simulink model "gm_ControllerTestbench"  (R2020b)
settings: Solver=VariableStepAuto  StartTime=0.0  StopTime=4  RelTol=1e-3
model workspace (MAT data in the model file):
  randSeedTorque = 0
  randomSeedSpeed = 0
undefined symbols (not defined in the file or in its folder): DiscIntNeverNeededParam, I_max, Position_PI_Limit
libraries: simulink x4, hdlmdlgenlib x1
(part 1 of 2)
settings Model: Creator=ciaran  LastModifiedBy=ciaran
settings OptimizationCC: BlockReduction=off  ConditionallyExecuteInputs=off
settings DebuggingCC: InheritedTsInSrcMsg=none

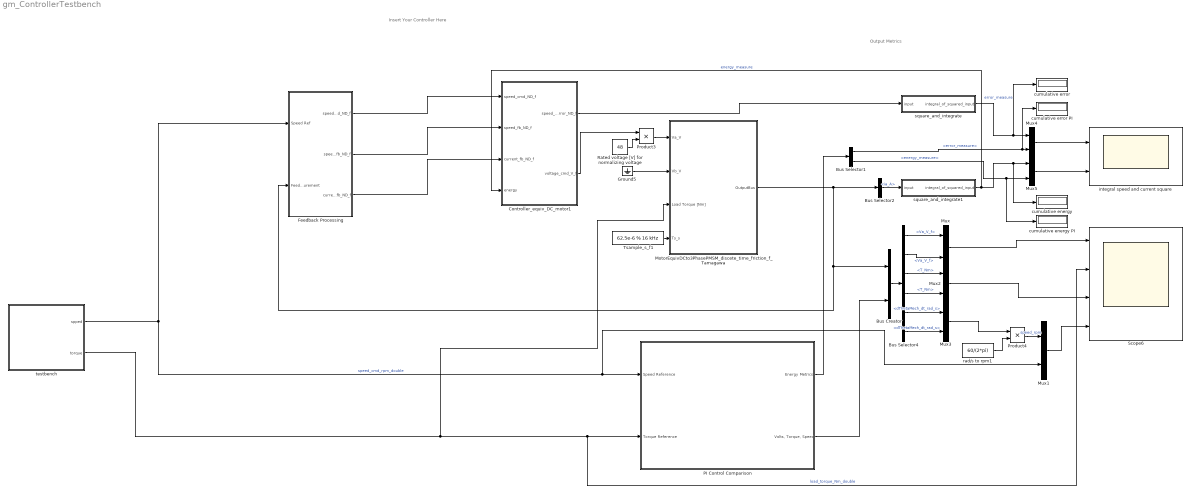
== system gm_ControllerTestbench ==
  note: Insert Your Controller Here
  note: Output Metrics
  Bus Creator : BusCreator  Inputs=2
  Bus Selector1 : BusSelector  OutputSignals=error_measure,energy_measure
  Bus Selector2 : BusSelector  OutputSignals=ia_A
  Bus Selector4 : BusSelector  OutputSignals=signal1.Va_V_f,signal2.Va_V_f,signal1.T_Nm,signal2.T_Nm,signal1.dThetaMech_dt_rad_s,signal2.dThetaMech_dt_rad_s
  Controller_equiv_DC_motor1 : Subsystem
  Feedback Processing : Subsystem
  Ground5 : Ground
  MotorEquivDCto3PhasePMSM_discete_time_friction_f_Tamagawa : Subsystem  mask(Intel PMSM equiv DC){R_ohm=0.68/3, L_H=3e-3/3, Ke_Vs_rad=0.07, Kt_Nm_A=0.07, PolePairs_int=2, J_kgm2=0.165e-4, Tf_Nm=0.02}
      mask prompts: R_ohm "Phase resistance [Ohm]"; L_H "Phase inductance [H]"; Ke_Vs_rad "Back-emf constant kE, based on peak phase values [Vs/rad]"; Kt_Nm_A "Motor torque constant kT, based on peak phase values [Nm/A]"; PolePairs_int "Number of pole pairs (0.5*n poles)  [integer]"; J_kgm2 "Mechanical inertia [kgm^2]"; Tf_Nm "Static friction Tf [Nm]"
      mask help: Intel motor model, equiv DC to PMSM
  Mux{,1..5} (6 alike) : Mux  Inputs=2
  PI Control Comparison : Subsystem
  Product3 : Product
  Product4 : Product
  Rated voltage [V] for normalizing voltage : Constant  Value=48  OutDataTypeStr=double
  Scope6 : Scope  NumInputPorts=4
  Tsample_s_f1 : Constant  Value=62.5e-6 % 16 kHz  OutDataTypeStr=double
  cumulative energy : Display
  cumulative energy PI : Display
  cumulative error : Display
  cumulative error PI : Display
  integral speed and current square : Scope  NumInputPorts=2
  rad/s to rpm1 : Constant  Value=60/(2*pi)  OutDataTypeStr=double
  square_and_integrate : Subsystem
  square_and_integrate1 : Subsystem
  testbench : Subsystem
  wires:
  Bus Selector2/1 -> square_and_integrate1/1(input)  "<ia_A>"
  Ground5/1 -> MotorEquivDCto3PhasePMSM_discete_time_friction_f_Tamagawa/2(Vb_V)
  Tsample_s_f1/1 -> MotorEquivDCto3PhasePMSM_discete_time_friction_f_Tamagawa/4(Ts_s)
  rad/s to rpm1/1 -> Product4/2
  square_and_integrate1/1(integral_of_squared_input) -> Controller_equiv_DC_motor1/4(energy), cumulative energy/1, Mux5/1  "energy_measure"
  Controller_equiv_DC_motor1/1(speed_error_ND_f) -> square_and_integrate/1(input)
  MotorEquivDCto3PhasePMSM_discete_time_friction_f_Tamagawa/1(OutputBus) -> Feedback Processing/2(Feedback Measurement), Bus Creator/1, Bus Selector2/1
  square_and_integrate/1(integral_of_squared_input) -> Mux4/1, cumulative error/1  "error_measure"
  testbench/1(spped) -> Mux1/2, PI Control Comparison/1(Speed Reference), Feedback Processing/1(Speed Ref)  "speed_cmd_rpm_double"
  testbench/2(torque) -> MotorEquivDCto3PhasePMSM_discete_time_friction_f_Tamagawa/3(Load Torque [Nm]), Scope6/2, PI Control Comparison/2(Torque Reference)  "load_torque_Nm_double"
  Feedback Processing/1(speed_cmd_ND_f) -> Controller_equiv_DC_motor1/1(speed_cmd_ND_f)
  Feedback Processing/2(speed_fb_ND_f) -> Controller_equiv_DC_motor1/2(speed_fb_ND_f)
  Feedback Processing/3(current_fb_ND_f) -> Controller_equiv_DC_motor1/3(current_fb_ND_f)
  PI Control Comparison/2("Volts, Torque, Speed") -> Bus Creator/2
  Bus Creator/1 -> Bus Selector4/1
  Bus Selector4/1 -> Mux/1  "<Va_V_f>"
  Bus Selector4/2 -> Mux/2  "<Va_V_f>"
  Bus Selector4/3 -> Mux2/1  "<T_Nm>"
  Bus Selector4/4 -> Mux2/2  "<T_Nm>"
  Mux2/1 -> Scope6/3
  Mux3/1 -> Product4/1
  PI Control Comparison/1(Energy Metrics) -> Bus Selector1/1
  Mux4/1 -> integral speed and current square/1
  Bus Selector1/1 -> cumulative error PI/1, Mux4/2  "<error_measure>"
  Mux5/1 -> integral speed and current square/2
  Bus Selector1/2 -> cumulative energy PI/1, Mux5/2  "<energy_measure>"
  Rated voltage [V] for normalizing voltage/1 -> Product3/2
  Controller_equiv_DC_motor1/2(voltage_cmd_V_f) -> Product3/1
  Product3/1 -> MotorEquivDCto3PhasePMSM_discete_time_friction_f_Tamagawa/1(Va_V)
  Product4/1 -> Mux1/1  "speed_rpm"
  Mux1/1 -> Scope6/4
  Mux/1 -> Scope6/1
  Bus Selector4/5 -> Mux3/1  "<dThetaMech_dt_rad_s>"
  Bus Selector4/6 -> Mux3/2  "<dThetaMech_dt_rad_s>"

== system gm_ControllerTestbench/Controller_equiv_DC_motor1 ==
  note: RL Controller
  speed_cmd_ND_f : Inport
  speed_fb_ND_f : Inport  Port=2  PortDimensions=1
  current_fb_ND_f : Inport  Port=3  PortDimensions=1
  energy : Inport  Port=4
  1 to reset : ManualSwitch
  FALSE_bool : Constant  Value=0  OutDataTypeStr=boolean
  PI_Ctrl_float_speed : Subsystem
  TRUE_bool : Constant  OutDataTypeStr=boolean
  abs_limit_output_ND_f : Constant  OutDataTypeStr=double
  speed_error_ND_f : Outport
  voltage_cmd_V_f : Outport  Port=2
  wires:
  speed_cmd_ND_f/1 -> PI_Ctrl_float_speed/1(cmd_f)
  speed_fb_ND_f/1 -> PI_Ctrl_float_speed/2(fb_f)
  abs_limit_output_ND_f/1 -> PI_Ctrl_float_speed/3(output_abs_limit_f)
  current_fb_ND_f/1 -> PI_Ctrl_float_speed/6(Icurrent_fb)
  1 to reset/1 -> PI_Ctrl_float_speed/4(Reset_bool)
  FALSE_bool/1 -> 1 to reset/1
  TRUE_bool/1 -> 1 to reset/2
  PI_Ctrl_float_speed/1(error_f) -> speed_error_ND_f/1  "speed_error_ND_f"
  energy/1 -> PI_Ctrl_float_speed/5(energy)
  PI_Ctrl_float_speed/2(output_f) -> voltage_cmd_V_f/1

== system gm_ControllerTestbench/Feedback Processing ==
  note: Constant Parameters
  note: Feedback Variables (Observations)
  Speed Ref : Inport
  Feedback Measurement : Inport  Port=2
  Bus Selector1 : BusSelector  OutputSignals=dThetaMech_dt_rad_s,ia_A
  Delay_current_measure : Delay  DelayLength=1  InitialCondition=0
  Delay_speed_measure : Delay  InitialCondition=0
  Inverse ated current [A] for normalizing current : Constant  Value=1/5.7  OutDataTypeStr=double
  Inverse rated speed [1/rpm] for normalizing speed : Constant  Value=1/5000  OutDataTypeStr=double
  Product : Product
  Product1 : Product  Inputs=***
  Product2 : Product
  rad/s to rpm : Constant  Value=60/(2*pi)  OutDataTypeStr=double
  speed_cmd_ND_f : Outport
  speed_fb_ND_f : Outport  Port=2
  current_fb_ND_f : Outport  Port=3
  wires:
  Speed Ref/1 -> Product/1
  Feedback Measurement/1 -> Bus Selector1/1
  Inverse ated current [A] for normalizing current/1 -> Product2/2  "speed_cmd_rpm_double"
  Delay_current_measure/1 -> current_fb_ND_f/1
  rad/s to rpm/1 -> Product1/2
  Product/1 -> speed_cmd_ND_f/1  "speed_cmd_ND_f"
  Product1/1 -> Delay_speed_measure/1  "speed_fb_ND_f"
  Bus Selector1/2 -> Product2/1  "<ia_A>"
  Bus Selector1/1 -> Product1/3  "<dThetaMech_dt_rad_s>"
  Delay_speed_measure/1 -> speed_fb_ND_f/1
  Product2/1 -> Delay_current_measure/1  "current_fb_ND_f"
  Inverse rated speed [1/rpm] for normalizing speed/1 -> Product1/1, Product/2

== system gm_ControllerTestbench/MotorEquivDCto3PhasePMSM_discete_time_friction_f_Tamagawa ==
  Va_V : Inport
  Vb_V : Inport  Port=2
  Load Torque [Nm] : Inport  Port=3
  Ts_s : Inport  Port=4
  Bus Creator1 : BusCreator  Inputs=7
  Load Torque [Nm]1 : InportShadow  Port=3
  Motor electromagnetic : Subsystem
  Motor mechanical : Subsystem  mask(Inertia){J_kgm2=J_kgm2}
      mask prompts: J_kgm2 "Inertia [kgm^2]"
      mask help:
      | Mechanical inertia with two attachment points A and B.
      | Torque is applied to the inertia from side A and side B.
      | The combined torque acting on the inertia produces acceleration,
      | velocity and displacement. Velocity and displacement are output as these
      | are the states of the system.
  Ts_s1 : InportShadow  Port=4
  Va_V1 : InportShadow
  Vb_V1 : InportShadow  Port=2
  OutputBus : Outport
  wires:
  Ts_s1/1 -> Motor electromagnetic/4(Ts_s)
  Motor mechanical/1(dTheta_dt_rad_s) -> Motor electromagnetic/3(dThetaMech_dt_rad_s), Bus Creator1/6  "dThetaMech_dt_rad_s"
  Ts_s/1 -> Motor mechanical/3(Ts_s)
  Load Torque [Nm]/1 -> Motor mechanical/2(TB_Nm)  "TL_Nm_f"
  Va_V/1 -> Motor electromagnetic/1(Va_V)  "Va_V_f"
  Bus Creator1/1 -> OutputBus/1
  Vb_V/1 -> Motor electromagnetic/2(Vb_V)  "Vb_V_f"
  Va_V1/1 -> Bus Creator1/1  "Va_V_f"
  Vb_V1/1 -> Bus Creator1/2  "Vb_V_f"
  Motor electromagnetic/1(ia_A) -> Bus Creator1/4  "ia_A"
  Motor electromagnetic/2(T_Nm) -> Motor mechanical/1(TA_Nm), Bus Creator1/5  "T_Nm"
  Motor mechanical/2(Theta_rad) -> Bus Creator1/7  "ThetaMech_rad"
  Load Torque [Nm]1/1 -> Bus Creator1/3  "TL_Nm_f"

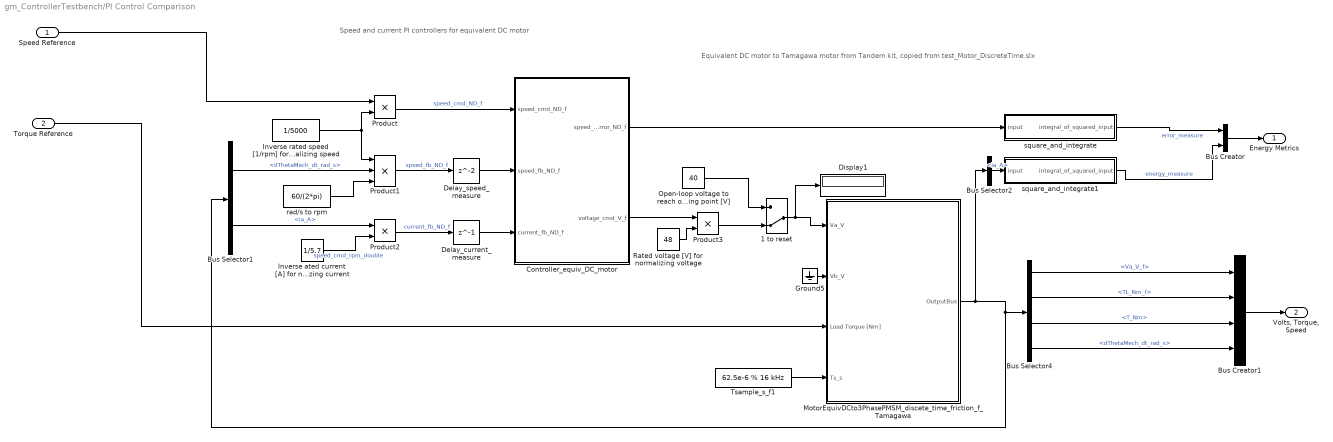
== system gm_ControllerTestbench/PI Control Comparison ==
  note: Speed and current PI controllers
      | for equivalent DC motor
  note: Equivalent DC motor to Tamagawa motor from Tandem kit,
      | copied from test_Motor_DiscreteTime.slx
  Speed Reference : Inport
  Torque Reference : Inport  Port=2
  1 to reset : ManualSwitch  CurrentSetting=0
  Bus Creator : BusCreator  Inputs=2
  Bus Creator1 : BusCreator  Inputs=4
  Bus Selector1 : BusSelector  OutputSignals=dThetaMech_dt_rad_s,ia_A
  Bus Selector2 : BusSelector  OutputSignals=ia_A
  Bus Selector4 : BusSelector  OutputSignals=Va_V_f,TL_Nm_f,T_Nm,dThetaMech_dt_rad_s
  Controller_equiv_DC_motor : Subsystem
  Delay_current_measure : Delay  DelayLength=1  InitialCondition=0
  Delay_speed_measure : Delay  InitialCondition=0
  Display1 : Display
  Ground5 : Ground
  Inverse ated current [A] for normalizing current : Constant  Value=1/5.7  OutDataTypeStr=double
  Inverse rated speed [1/rpm] for normalizing speed : Constant  Value=1/5000  OutDataTypeStr=double
  MotorEquivDCto3PhasePMSM_discete_time_friction_f_Tamagawa : Subsystem  mask(Intel PMSM equiv DC){R_ohm=0.68/3, L_H=3e-3/3, Ke_Vs_rad=0.07, Kt_Nm_A=0.07, PolePairs_int=2, J_kgm2=0.165e-4, Tf_Nm=0.02}
      mask prompts: R_ohm "Phase resistance [Ohm]"; L_H "Phase inductance [H]"; Ke_Vs_rad "Back-emf constant kE, based on peak phase values [Vs/rad]"; Kt_Nm_A "Motor torque constant kT, based on peak phase values [Nm/A]"; PolePairs_int "Number of pole pairs (0.5*n poles)  [integer]"; J_kgm2 "Mechanical inertia [kgm^2]"; Tf_Nm "Static friction Tf [Nm]"
      mask help: Intel motor model, equiv DC to PMSM
  Open-loop voltage to reach operating point [V] : Constant  Value=40  OutDataTypeStr=double
  Product : Product
  Product1 : Product  Inputs=***
  Product2 : Product
  Product3 : Product
  Rated voltage [V] for normalizing voltage : Constant  Value=48  OutDataTypeStr=double
  Tsample_s_f1 : Constant  Value=62.5e-6 % 16 kHz  OutDataTypeStr=double
  rad/s to rpm : Constant  Value=60/(2*pi)  OutDataTypeStr=double
  square_and_integrate : Subsystem
  square_and_integrate1 : Subsystem
  Energy Metrics : Outport
  "Volts, Torque, Speed" : Outport  Port=2
  wires:
  Open-loop voltage to reach operating point [V]/1 -> 1 to reset/1
  Delay_speed_measure/1 -> Controller_equiv_DC_motor/2(speed_fb_ND_f)
  Ground5/1 -> MotorEquivDCto3PhasePMSM_discete_time_friction_f_Tamagawa/2(Vb_V)
  Tsample_s_f1/1 -> MotorEquivDCto3PhasePMSM_discete_time_friction_f_Tamagawa/4(Ts_s)
  Controller_equiv_DC_motor/2(voltage_cmd_V_f) -> Product3/1
  Inverse ated current [A] for normalizing current/1 -> Product2/2  "speed_cmd_rpm_double"
  Controller_equiv_DC_motor/1(speed_error_ND_f) -> square_and_integrate/1(input)
  Rated voltage [V] for normalizing voltage/1 -> Product3/2
  square_and_integrate1/1(integral_of_squared_input) -> Bus Creator/2  "energy_measure"
  Bus Selector1/2 -> Product2/1  "<ia_A>"
  Delay_current_measure/1 -> Controller_equiv_DC_motor/3(current_fb_ND_f)
  Bus Selector1/1 -> Product1/2  "<dThetaMech_dt_rad_s>"
  rad/s to rpm/1 -> Product1/3
  Product2/1 -> Delay_current_measure/1  "current_fb_ND_f"
  Product3/1 -> 1 to reset/2
  Bus Selector2/1 -> square_and_integrate1/1(input)  "<ia_A>"
  Inverse rated speed [1/rpm] for normalizing speed/1 -> Product/2, Product1/1
  MotorEquivDCto3PhasePMSM_discete_time_friction_f_Tamagawa/1(OutputBus) -> Bus Selector2/1, Bus Selector1/1, Bus Selector4/1
  1 to reset/1 -> Display1/1, MotorEquivDCto3PhasePMSM_discete_time_friction_f_Tamagawa/1(Va_V)
  Product1/1 -> Delay_speed_measure/1  "speed_fb_ND_f"
  Product/1 -> Controller_equiv_DC_motor/1(speed_cmd_ND_f)  "speed_cmd_ND_f"
  square_and_integrate/1(integral_of_squared_input) -> Bus Creator/1  "error_measure"
  Torque Reference/1 -> MotorEquivDCto3PhasePMSM_discete_time_friction_f_Tamagawa/3(Load Torque [Nm])
  Speed Reference/1 -> Product/1
  Bus Selector4/1 -> Bus Creator1/1  "<Va_V_f>"
  Bus Selector4/2 -> Bus Creator1/2  "<TL_Nm_f>"
  Bus Selector4/3 -> Bus Creator1/3  "<T_Nm>"
  Bus Selector4/4 -> Bus Creator1/4  "<dThetaMech_dt_rad_s>"
  Bus Creator/1 -> Energy Metrics/1
  Bus Creator1/1 -> "Volts, Torque, Speed"/1

== system gm_ControllerTestbench/square_and_integrate ==
  input : Inport
  Add : Sum
  Product6 : Product  Inputs=***
  Tsample_s_f2 : Constant  Value=62.5e-6 % 16 kHz  OutDataTypeStr=double
  delay_to_integrate : Delay  DelayLength=1  InitialCondition=0
  integral_of_squared_input : Outport
  wires:
  delay_to_integrate/1 -> integral_of_squared_input/1, Add/2
  Product6/1 -> Add/1
  Tsample_s_f2/1 -> Product6/3
  Add/1 -> delay_to_integrate/1
  input/1 -> Product6/1, Product6/2

== system gm_ControllerTestbench/square_and_integrate1 ==
  input : Inport
  Add : Sum
  Product6 : Product  Inputs=***
  Tsample_s_f2 : Constant  Value=62.5e-6 % 16 kHz  OutDataTypeStr=double
  delay_to_integrate : Delay  DelayLength=1  InitialCondition=0
  integral_of_squared_input : Outport
  wires:
  input/1 -> Product6/2, Product6/1
  Add/1 -> delay_to_integrate/1
  Tsample_s_f2/1 -> Product6/3
  Product6/1 -> Add/1
  delay_to_integrate/1 -> Add/2, integral_of_squared_input/1

== system gm_ControllerTestbench/testbench ==
  Constant : Constant  Value=5000
  Gain : Gain  Gain=0.38
  Rate Transition2 : RateTransition  OutPortSampleTime=62.5e-6
  Rate Transition3 : RateTransition  OutPortSampleTime=62.5e-6
  Repeating Sequence Stair : simulink/Sources/Repeating Sequence Stair  OutValues="[5000 -5000 5000 0  0 100 0 -100 -1500 1500 200 -200 3000 -3000 -4000 4000 0 10 20 0 -10 -20].'"  tsamp=3500*62.5e-6  OutMin=[]  OutMax=[]  OutDataTypeStr=double  OutputDataTypeScalingMode=double  OutDataType=fixdt(0,8)  ConRadixGroup=Best Precision: Vector-wise  OutScaling=2^-12
  Repeating Sequence Stair1 : simulink/Sources/Repeating Sequence Stair  OutValues=[1 -1 0 0.5 -0.5].'  tsamp=875*62.5e-6  OutMin=[]  OutMax=[]  OutDataTypeStr=double  OutputDataTypeScalingMode=double  OutDataType=fixdt(0,8)  ConRadixGroup=Best Precision: Vector-wise  OutScaling=2^-12
  spped : Outport
  torque : Outport  Port=2
  wires:
  Rate Transition3/1 -> torque/1  "speed_cmd_rpm_double"
  Repeating Sequence Stair/1 -> Rate Transition2/1
  Repeating Sequence Stair1/1 -> Gain/1
  Gain/1 -> Rate Transition3/1
  Constant/1 -> spped/1

== system gm_ControllerTestbench/Controller_equiv_DC_motor1/PI_Ctrl_float_speed ==
  note: Error Input
  cmd_f : Inport
  fb_f : Inport  Port=2
  output_abs_limit_f : Inport  Port=3
  Reset_bool : Inport  Port=4
  energy : Inport  Port=5
  Icurrent_fb : Inport  Port=6
  Constant1 : Constant  Value=0  OutDataTypeStr=Inherit: Inherit via back propagation
  Reinforcement Learning1 : Subsystem
  Subtract1 : Sum  Inputs=+-
  Unit Delay1 : UnitDelay  SampleTime=-1  HasFrameUpgradeWarning=on
  limit_abs_value_of_output : Subsystem
  set_output_to_zero_if_reset : Switch  Criteria=u2 > Threshold
  error_f : Outport
  output_f : Outport  Port=2
  wires:
  output_abs_limit_f/1 -> Reinforcement Learning1/7(abslimit), limit_abs_value_of_output/2(abs_max)
  limit_abs_value_of_output/1(output) -> Unit Delay1/1, set_output_to_zero_if_reset/3
  set_output_to_zero_if_reset/1 -> output_f/1
  Reset_bool/1 -> Reinforcement Learning1/2(isdone), set_output_to_zero_if_reset/2
  Constant1/1 -> set_output_to_zero_if_reset/1
  cmd_f/1 -> Reinforcement Learning1/8(speedin), Subtract1/1
  fb_f/1 -> Subtract1/2, Reinforcement Learning1/4(speedfb)
  Subtract1/1 -> Reinforcement Learning1/1(speederror), error_f/1  "error_f"
  energy/1 -> Reinforcement Learning1/3(energy measure)
  Icurrent_fb/1 -> Reinforcement Learning1/5(cfb)
  Unit Delay1/1 -> Reinforcement Learning1/6(prevact)
  Reinforcement Learning1/1(action) -> limit_abs_value_of_output/1(input)

== system gm_ControllerTestbench/MotorEquivDCto3PhasePMSM_discete_time_friction_f_Tamagawa/Motor electromagnetic ==
  note: Single phase to get same rated operating point as 3-phase
  note: Calculate current in phase a.
  Va_V : Inport
  Vb_V : Inport  Port=2
  dThetaMech_dt_rad_s : Inport  Port=3
  Ts_s : Inport  Port=4
  Delay : Delay  DelayLength=1
  Gain_Kt_Nm_A : Gain  Gain=Kt_Nm_A
  Ke_Vs_rad : Gain  Gain=Ke_Vs_rad
  Product : Product
  Sum : Sum  Inputs=|++
  Sum6 : Sum  Inputs=+---
  gain_Ra : Gain  Gain=3*R_ohm
  gain_inverseInductance : Gain  Gain=1/(3*L_H)
  ia_A : Outport
  T_Nm : Outport  Port=2
  wires:
  Ts_s/1 -> Product/2
  Sum/1 -> Delay/1
  Product/1 -> Sum/1
  Delay/1 -> gain_Ra/1, Sum/2, Gain_Kt_Nm_A/1, ia_A/1  "ia_A"
  gain_Ra/1 -> Sum6/4
  gain_inverseInductance/1 -> Product/1  "dia/dt"
  Ke_Vs_rad/1 -> Sum6/3
  Sum6/1 -> gain_inverseInductance/1  "vLa_V"
  Vb_V/1 -> Sum6/2
  dThetaMech_dt_rad_s/1 -> Ke_Vs_rad/1  "dThetaMech_dt_rad_s"
  Gain_Kt_Nm_A/1 -> T_Nm/1  "T_Nm"
  Va_V/1 -> Sum6/1

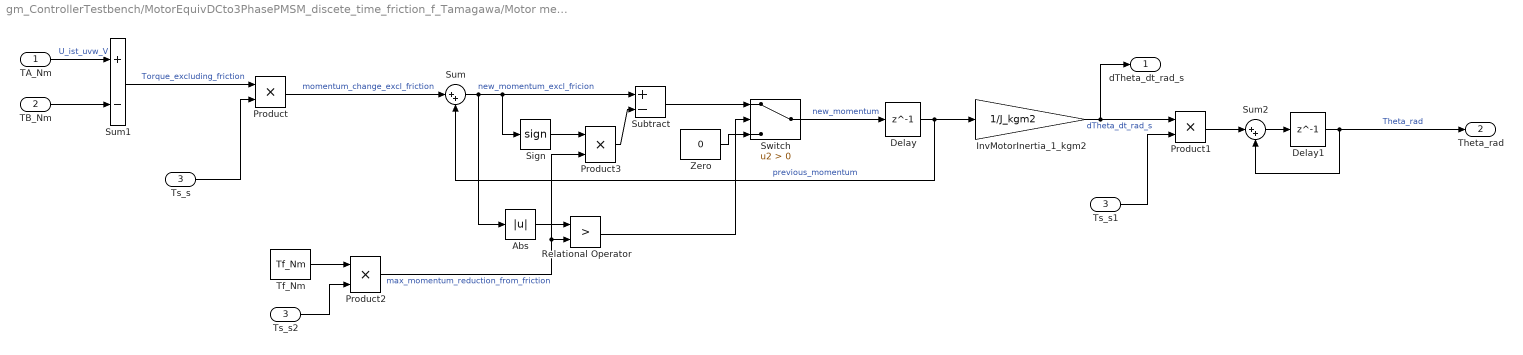
== system gm_ControllerTestbench/MotorEquivDCto3PhasePMSM_discete_time_friction_f_Tamagawa/Motor mechanical ==
  TA_Nm : Inport
  TB_Nm : Inport  Port=2
  Ts_s : Inport  Port=3
  Abs : Abs
  Delay : Delay  DelayLength=1
  Delay1 : Delay  DelayLength=1
  InvMotorInertia_1_kgm2 : Gain  Gain=1/J_kgm2
  Product{,1..3} (4 alike) : Product
  Relational Operator : RelationalOperator  Operator=>  OutDataTypeStr=boolean  RndMeth=Nearest
  Sign : Signum
  Subtract : Sum  Inputs=+-
  Sum : Sum  Inputs=|++
  Sum1 : Sum  Inputs=+-
  Sum2 : Sum  Inputs=|++
  Switch : Switch  Criteria=u2 > Threshold
  Tf_Nm : Constant  Value=Tf_Nm
  Ts_s1 : InportShadow  Port=3
  Ts_s2 : InportShadow  Port=3
  Zero : Constant  Value=0
  dTheta_dt_rad_s : Outport
  Theta_rad : Outport  Port=2
  wires:
  Product1/1 -> Sum2/1
  Sum2/1 -> Delay1/1
  Delay1/1 -> Theta_rad/1, Sum2/2  "Theta_rad"
  Sum/1 -> Abs/1, Sign/1, Subtract/1  "new_momentum_excl_fricion"
  Product/1 -> Sum/1  "momentum_change_excl_friction"
  Ts_s/1 -> Product/2
  Sum1/1 -> Product/1  "Torque_excluding_friction"
  TB_Nm/1 -> Sum1/2
  TA_Nm/1 -> Sum1/1  "U_ist_uvw_V"
  Ts_s1/1 -> Product1/2
  Delay/1 -> InvMotorInertia_1_kgm2/1, Sum/2  "previous_momentum"
  Tf_Nm/1 -> Product2/1
  Ts_s2/1 -> Product2/2
  Product2/1 -> Product3/2, Relational Operator/2  "max_momentum_reduction_from_friction"
  Abs/1 -> Relational Operator/1
  Relational Operator/1 -> Switch/2
  Sign/1 -> Product3/1
  Product3/1 -> Subtract/2
  Subtract/1 -> Switch/1
  Zero/1 -> Switch/3
  Switch/1 -> Delay/1  "new_momentum"
  InvMotorInertia_1_kgm2/1 -> dTheta_dt_rad_s/1, Product1/1  "dTheta_dt_rad_s"

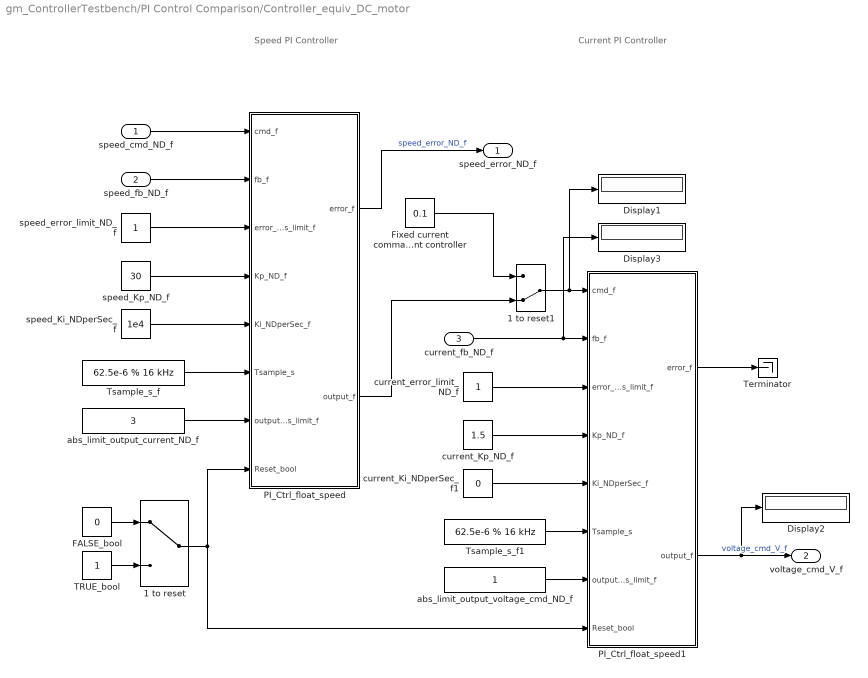
== system gm_ControllerTestbench/PI Control Comparison/Controller_equiv_DC_motor ==
  note: Speed
      | PI Controller
  note: Current
      | PI Controller
  speed_cmd_ND_f : Inport
  speed_fb_ND_f : Inport  Port=2  PortDimensions=1
  current_fb_ND_f : Inport  Port=3  PortDimensions=1
  1 to reset : ManualSwitch
  1 to reset1 : ManualSwitch  CurrentSetting=0
  Display1 : Display
  Display2 : Display
  Display3 : Display
  FALSE_bool : Constant  Value=0  OutDataTypeStr=boolean
  Fixed current command for tuning current controller : Constant  Value=0.1  OutDataTypeStr=double
  PI_Ctrl_float_speed : Subsystem
  PI_Ctrl_float_speed1 : Subsystem
  TRUE_bool : Constant  OutDataTypeStr=boolean
  Terminator : Terminator
  Tsample_s_f : Constant  Value=62.5e-6 % 16 kHz  OutDataTypeStr=double
  Tsample_s_f1 : Constant  Value=62.5e-6 % 16 kHz  OutDataTypeStr=double
  abs_limit_output_current_ND_f : Constant  Value=3  OutDataTypeStr=double
  abs_limit_output_voltage_cmd_ND_f : Constant  OutDataTypeStr=double
  current_Ki_NDperSec_f1 : Constant  Value=0  OutDataTypeStr=double
  current_Kp_ND_f : Constant  Value=1.5  OutDataTypeStr=double
  current_error_limit_ND_f : Constant  OutDataTypeStr=double
  speed_Ki_NDperSec_f : Constant  Value=1e4  OutDataTypeStr=double
  speed_Kp_ND_f : Constant  Value=30  OutDataTypeStr=double
  speed_error_limit_ND_f : Constant  OutDataTypeStr=double
  speed_error_ND_f : Outport
  voltage_cmd_V_f : Outport  Port=2
  wires:
  speed_cmd_ND_f/1 -> PI_Ctrl_float_speed/1(cmd_f)
  speed_fb_ND_f/1 -> PI_Ctrl_float_speed/2(fb_f)
  speed_error_limit_ND_f/1 -> PI_Ctrl_float_speed/3(error_abs_limit_f)
  speed_Kp_ND_f/1 -> PI_Ctrl_float_speed/4(Kp_ND_f)
  speed_Ki_NDperSec_f/1 -> PI_Ctrl_float_speed/5(Ki_NDperSec_f)
  Tsample_s_f/1 -> PI_Ctrl_float_speed/6(Tsample_s)
  abs_limit_output_current_ND_f/1 -> PI_Ctrl_float_speed/7(output_abs_limit_f)
  current_fb_ND_f/1 -> PI_Ctrl_float_speed1/2(fb_f), Display3/1
  Tsample_s_f1/1 -> PI_Ctrl_float_speed1/6(Tsample_s)
  current_error_limit_ND_f/1 -> PI_Ctrl_float_speed1/3(error_abs_limit_f)
  current_Kp_ND_f/1 -> PI_Ctrl_float_speed1/4(Kp_ND_f)
  current_Ki_NDperSec_f1/1 -> PI_Ctrl_float_speed1/5(Ki_NDperSec_f)
  abs_limit_output_voltage_cmd_ND_f/1 -> PI_Ctrl_float_speed1/7(output_abs_limit_f)
  1 to reset/1 -> PI_Ctrl_float_speed1/8(Reset_bool), PI_Ctrl_float_speed/8(Reset_bool)
  PI_Ctrl_float_speed1/2(output_f) -> Display2/1, voltage_cmd_V_f/1  "voltage_cmd_V_f"
  FALSE_bool/1 -> 1 to reset/1
  TRUE_bool/1 -> 1 to reset/2
  PI_Ctrl_float_speed/2(output_f) -> 1 to reset1/2
  Fixed current command for tuning current controller/1 -> 1 to reset1/1
  1 to reset1/1 -> PI_Ctrl_float_speed1/1(cmd_f), Display1/1
  PI_Ctrl_float_speed/1(error_f) -> speed_error_ND_f/1  "speed_error_ND_f"
  PI_Ctrl_float_speed1/1(error_f) -> Terminator/1

== system gm_ControllerTestbench/PI Control Comparison/MotorEquivDCto3PhasePMSM_discete_time_friction_f_Tamagawa ==
  Va_V : Inport
  Vb_V : Inport  Port=2
  Load Torque [Nm] : Inport  Port=3
  Ts_s : Inport  Port=4
  Bus Creator1 : BusCreator  Inputs=7
  Load Torque [Nm]1 : InportShadow  Port=3
  Motor electromagnetic : Subsystem
  Motor mechanical : Subsystem  mask(Inertia){J_kgm2=J_kgm2}
      mask prompts: J_kgm2 "Inertia [kgm^2]"
      mask help:
      | Mechanical inertia with two attachment points A and B.
      | Torque is applied to the inertia from side A and side B.
      | The combined torque acting on the inertia produces acceleration,
      | velocity and displacement. Velocity and displacement are output as these
      | are the states of the system.
  Ts_s1 : InportShadow  Port=4
  Va_V1 : InportShadow
  Vb_V1 : InportShadow  Port=2
  OutputBus : Outport
  wires:
  Ts_s1/1 -> Motor electromagnetic/4(Ts_s)
  Motor mechanical/1(dTheta_dt_rad_s) -> Motor electromagnetic/3(dThetaMech_dt_rad_s), Bus Creator1/6  "dThetaMech_dt_rad_s"
  Ts_s/1 -> Motor mechanical/3(Ts_s)
  Load Torque [Nm]/1 -> Motor mechanical/2(TB_Nm)  "TL_Nm_f"
  Va_V/1 -> Motor electromagnetic/1(Va_V)  "Va_V_f"
  Bus Creator1/1 -> OutputBus/1
  Vb_V/1 -> Motor electromagnetic/2(Vb_V)  "Vb_V_f"
  Va_V1/1 -> Bus Creator1/1  "Va_V_f"
  Vb_V1/1 -> Bus Creator1/2  "Vb_V_f"
  Motor electromagnetic/1(ia_A) -> Bus Creator1/4  "ia_A"
  Motor electromagnetic/2(T_Nm) -> Motor mechanical/1(TA_Nm), Bus Creator1/5  "T_Nm"
  Motor mechanical/2(Theta_rad) -> Bus Creator1/7  "ThetaMech_rad"
  Load Torque [Nm]1/1 -> Bus Creator1/3  "TL_Nm_f"

== system gm_ControllerTestbench/PI Control Comparison/square_and_integrate ==
  input : Inport
  Add : Sum
  Product6 : Product  Inputs=***
  Tsample_s_f2 : Constant  Value=62.5e-6 % 16 kHz  OutDataTypeStr=double
  delay_to_integrate : Delay  DelayLength=1  InitialCondition=0
  integral_of_squared_input : Outport
  wires:
  delay_to_integrate/1 -> integral_of_squared_input/1, Add/2
  Product6/1 -> Add/1
  Tsample_s_f2/1 -> Product6/3
  Add/1 -> delay_to_integrate/1
  input/1 -> Product6/1, Product6/2

== system gm_ControllerTestbench/PI Control Comparison/square_and_integrate1 ==
  input : Inport
  Add : Sum
  Product6 : Product  Inputs=***
  Tsample_s_f2 : Constant  Value=62.5e-6 % 16 kHz  OutDataTypeStr=double
  delay_to_integrate : Delay  DelayLength=1  InitialCondition=0
  integral_of_squared_input : Outport
  wires:
  input/1 -> Product6/2, Product6/1
  Add/1 -> delay_to_integrate/1
  Tsample_s_f2/1 -> Product6/3
  Product6/1 -> Add/1
  delay_to_integrate/1 -> Add/2, integral_of_squared_input/1

== system gm_ControllerTestbench/Controller_equiv_DC_motor1/PI_Ctrl_float_speed/Reinforcement Learning1 ==
  speederror : Inport
  isdone : Inport  Port=2
  energy measure : Inport  Port=3
  speedfb : Inport  Port=4
  cfb : Inport  Port=5
  prevact : Inport  Port=6
  abslimit : Inport  Port=7
  speedin : Inport  Port=8
  Abs : Abs
  Add : Sum
  Data Type Conversion : DataTypeConversion
  Data Type Conversion1 : DataTypeConversion
  Delay : Delay  DelayLength=1
  GreaterThan : RelationalOperator  Operator=>  OutDataTypeStr=boolean  RndMeth=Simplest
  Multiply : Gain
  Observations : Subsystem
  Reward : Subsystem
  Subsystem Reference2 : Subsystem
  Unit Delay : UnitDelay  SampleTime=-1  HasFrameUpgradeWarning=on
  action : Outport
  wires:
  Data Type Conversion1/1 -> Add/1, Unit Delay/1
  Data Type Conversion/1 -> Subsystem Reference2/1(Observations)
  Observations/1(observations) -> Data Type Conversion/1
  Subsystem Reference2/1(Action) -> Data Type Conversion1/1
  prevact/1 -> Multiply/1
  Unit Delay/1 -> Reward/3(In3)
  Multiply/1 -> Add/2
  speedin/1 -> Observations/5(speedin)
  GreaterThan/1 -> Observations/4(lim)
  Abs/1 -> GreaterThan/1
  abslimit/1 -> GreaterThan/2
  Delay/1 -> Abs/1, Observations/6(prevact)
  Add/1 -> Delay/1, action/1
  cfb/1 -> Observations/3(curfb)
  speedfb/1 -> Observations/2(speedfb)
  energy measure/1 -> Reward/4(energy measure)
  speederror/1 -> Observations/1(speed err), Reward/2(error measure)
  isdone/1 -> Reward/1(done)

== system gm_ControllerTestbench/Controller_equiv_DC_motor1/PI_Ctrl_float_speed/limit_abs_value_of_output ==
  input : Inport
  abs_max : Inport  Port=2
  CmpLT : RelationalOperator  Operator=<  OutDataTypeStr=boolean  RndMeth=Nearest
  CmpLT1 : RelationalOperator  OutDataTypeStr=boolean  RndMeth=Nearest
  Switch : Switch  Criteria=u2 ~= 0  Threshold=Position_PI_Limit  ZeroCross=off
  Switch1 : Switch  Criteria=u2 ~= 0  Threshold=I_max  ZeroCross=off
  Unary Minus : UnaryMinus
  output : Outport
  wires:
  Unary Minus/1 -> CmpLT/2, Switch1/1
  Switch1/1 -> output/1
  Switch/1 -> Switch1/3
  CmpLT/1 -> Switch1/2
  input/1 -> CmpLT/1, Switch/3, CmpLT1/1
  abs_max/1 -> Unary Minus/1, CmpLT1/2, Switch/1
  CmpLT1/1 -> Switch/2

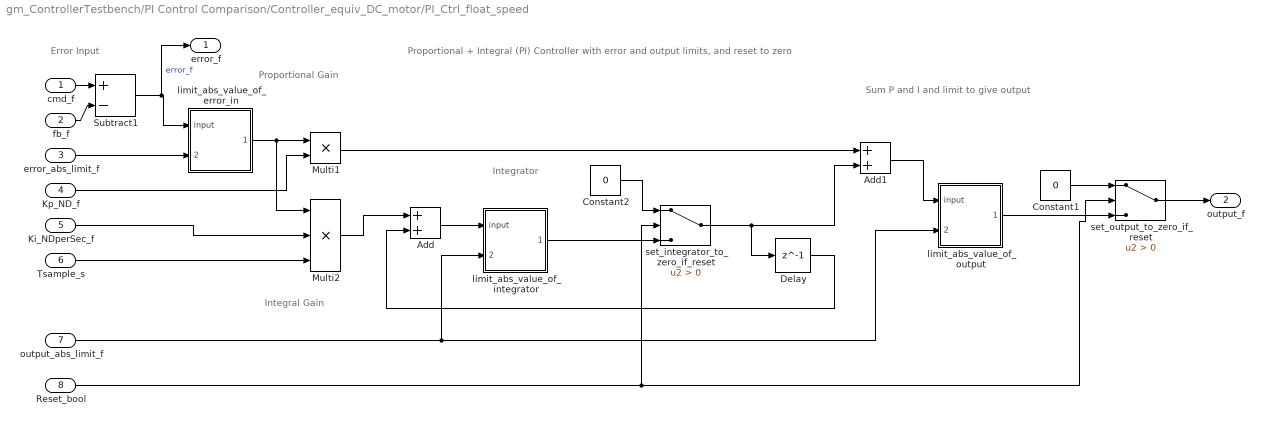
== system gm_ControllerTestbench/PI Control Comparison/Controller_equiv_DC_motor/PI_Ctrl_float_speed ==
  note: Proportional + Integral (PI) Controller with error and output limits, and reset to zero
  note: Error Input
  note: Proportional Gain
  note: Integral Gain
  note: Integrator
  note: Sum P and I and limit to give output
  cmd_f : Inport
  fb_f : Inport  Port=2
  error_abs_limit_f : Inport  Port=3
  Kp_ND_f : Inport  Port=4
  Ki_NDperSec_f : Inport  Port=5
  Tsample_s : Inport  Port=6
  output_abs_limit_f : Inport  Port=7
  Reset_bool : Inport  Port=8
  Add : Sum
  Add1 : Sum
  Constant1 : Constant  Value=0  OutDataTypeStr=Inherit: Inherit via back propagation
  Constant2 : Constant  Value=0  OutDataTypeStr=Inherit: Inherit via back propagation
  Delay : Delay  DelayLength=1  InitialCondition=0
  Multi1 : Product  Inputs=**  RndMeth=Zero  SaturateOnIntegerOverflow=on
  Multi2 : Product  Inputs=***  RndMeth=Zero  SaturateOnIntegerOverflow=on
  Subtract1 : Sum  Inputs=+-
  limit_abs_value_of_error_in : Subsystem
  limit_abs_value_of_integrator : Subsystem
  limit_abs_value_of_output : Subsystem
  set_integrator_to_zero_if_reset : Switch  Criteria=u2 > Threshold
  set_output_to_zero_if_reset : Switch  Criteria=u2 > Threshold
  error_f : Outport
  output_f : Outport  Port=2
  wires:
  Ki_NDperSec_f/1 -> Multi2/2
  Kp_ND_f/1 -> Multi1/2
  Delay/1 -> Add/2
  limit_abs_value_of_error_in/1(output) -> Multi1/1, Multi2/1
  error_abs_limit_f/1 -> limit_abs_value_of_error_in/2(abs_max)
  output_abs_limit_f/1 -> limit_abs_value_of_integrator/2(abs_max), limit_abs_value_of_output/2(abs_max)
  Multi1/1 -> Add1/1
  Multi2/1 -> Add/1
  Add/1 -> limit_abs_value_of_integrator/1(input)
  set_integrator_to_zero_if_reset/1 -> Add1/2, Delay/1
  Add1/1 -> limit_abs_value_of_output/1(input)
  limit_abs_value_of_output/1(output) -> set_output_to_zero_if_reset/3
  set_output_to_zero_if_reset/1 -> output_f/1
  Reset_bool/1 -> set_output_to_zero_if_reset/2, set_integrator_to_zero_if_reset/2
  Constant1/1 -> set_output_to_zero_if_reset/1
  Constant2/1 -> set_integrator_to_zero_if_reset/1
  limit_abs_value_of_integrator/1(output) -> set_integrator_to_zero_if_reset/3
  Tsample_s/1 -> Multi2/3
  cmd_f/1 -> Subtract1/1
  fb_f/1 -> Subtract1/2
  Subtract1/1 -> error_f/1, limit_abs_value_of_error_in/1(input)  "error_f"

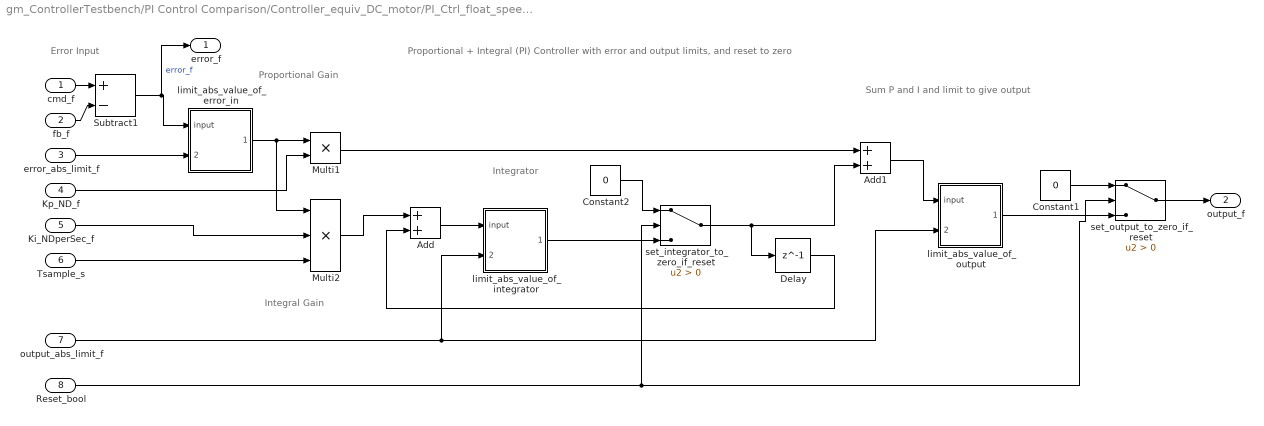
== system gm_ControllerTestbench/PI Control Comparison/Controller_equiv_DC_motor/PI_Ctrl_float_speed1 ==
  note: Sum P and I and limit to give output
  note: Integrator
  note: Integral Gain
  note: Proportional Gain
  note: Error Input
  note: Proportional + Integral (PI) Controller with error and output limits, and reset to zero
  cmd_f : Inport
  fb_f : Inport  Port=2
  error_abs_limit_f : Inport  Port=3
  Kp_ND_f : Inport  Port=4
  Ki_NDperSec_f : Inport  Port=5
  Tsample_s : Inport  Port=6
  output_abs_limit_f : Inport  Port=7
  Reset_bool : Inport  Port=8
  Add : Sum
  Add1 : Sum
  Constant1 : Constant  Value=0  OutDataTypeStr=Inherit: Inherit via back propagation
  Constant2 : Constant  Value=0  OutDataTypeStr=Inherit: Inherit via back propagation
  Delay : Delay  DelayLength=1  InitialCondition=0
  Multi1 : Product  Inputs=**  RndMeth=Zero  SaturateOnIntegerOverflow=on
  Multi2 : Product  Inputs=***  RndMeth=Zero  SaturateOnIntegerOverflow=on
  Subtract1 : Sum  Inputs=+-
  limit_abs_value_of_error_in : Subsystem
  limit_abs_value_of_integrator : Subsystem
  limit_abs_value_of_output : Subsystem
  set_integrator_to_zero_if_reset : Switch  Criteria=u2 > Threshold
  set_output_to_zero_if_reset : Switch  Criteria=u2 > Threshold
  error_f : Outport
  output_f : Outport  Port=2
  wires:
  Subtract1/1 -> limit_abs_value_of_error_in/1(input), error_f/1  "error_f"
  fb_f/1 -> Subtract1/2
  cmd_f/1 -> Subtract1/1
  Tsample_s/1 -> Multi2/3
  limit_abs_value_of_integrator/1(output) -> set_integrator_to_zero_if_reset/3
  Constant2/1 -> set_integrator_to_zero_if_reset/1
  Constant1/1 -> set_output_to_zero_if_reset/1
  Reset_bool/1 -> set_integrator_to_zero_if_reset/2, set_output_to_zero_if_reset/2
  set_output_to_zero_if_reset/1 -> output_f/1
  limit_abs_value_of_output/1(output) -> set_output_to_zero_if_reset/3
  Add1/1 -> limit_abs_value_of_output/1(input)
  set_integrator_to_zero_if_reset/1 -> Delay/1, Add1/2
  Add/1 -> limit_abs_value_of_integrator/1(input)
  Multi2/1 -> Add/1
  Multi1/1 -> Add1/1
  output_abs_limit_f/1 -> limit_abs_value_of_output/2(abs_max), limit_abs_value_of_integrator/2(abs_max)
  error_abs_limit_f/1 -> limit_abs_value_of_error_in/2(abs_max)
  limit_abs_value_of_error_in/1(output) -> Multi2/1, Multi1/1
  Delay/1 -> Add/2
  Kp_ND_f/1 -> Multi1/2
  Ki_NDperSec_f/1 -> Multi2/2

== system gm_ControllerTestbench/PI Control Comparison/MotorEquivDCto3PhasePMSM_discete_time_friction_f_Tamagawa/Motor electromagnetic ==
  note: Single phase to get same rated operating point as 3-phase
  note: Calculate current in phase a.
  Va_V : Inport
  Vb_V : Inport  Port=2
  dThetaMech_dt_rad_s : Inport  Port=3
  Ts_s : Inport  Port=4
  Delay : Delay  DelayLength=1
  Gain_Kt_Nm_A : Gain  Gain=Kt_Nm_A
  Ke_Vs_rad : Gain  Gain=Ke_Vs_rad
  Product : Product
  Sum : Sum  Inputs=|++
  Sum6 : Sum  Inputs=+---
  gain_Ra : Gain  Gain=3*R_ohm
  gain_inverseInductance : Gain  Gain=1/(3*L_H)
  ia_A : Outport
  T_Nm : Outport  Port=2
  wires:
  Ts_s/1 -> Product/2
  Sum/1 -> Delay/1
  Product/1 -> Sum/1
  Delay/1 -> gain_Ra/1, Sum/2, Gain_Kt_Nm_A/1, ia_A/1  "ia_A"
  gain_Ra/1 -> Sum6/4
  gain_inverseInductance/1 -> Product/1  "dia/dt"
  Ke_Vs_rad/1 -> Sum6/3
  Sum6/1 -> gain_inverseInductance/1  "vLa_V"
  Vb_V/1 -> Sum6/2
  dThetaMech_dt_rad_s/1 -> Ke_Vs_rad/1  "dThetaMech_dt_rad_s"
  Gain_Kt_Nm_A/1 -> T_Nm/1  "T_Nm"
  Va_V/1 -> Sum6/1

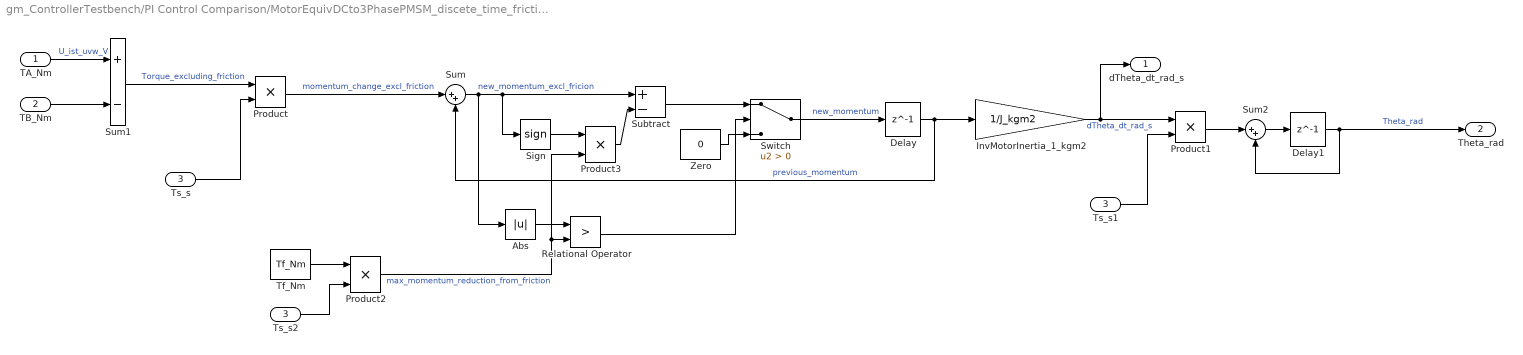
== system gm_ControllerTestbench/PI Control Comparison/MotorEquivDCto3PhasePMSM_discete_time_friction_f_Tamagawa/Motor mechanical ==
  TA_Nm : Inport
  TB_Nm : Inport  Port=2
  Ts_s : Inport  Port=3
  Abs : Abs
  Delay : Delay  DelayLength=1
  Delay1 : Delay  DelayLength=1
  InvMotorInertia_1_kgm2 : Gain  Gain=1/J_kgm2
  Product{,1..3} (4 alike) : Product
  Relational Operator : RelationalOperator  Operator=>  OutDataTypeStr=boolean  RndMeth=Nearest
  Sign : Signum
  Subtract : Sum  Inputs=+-
  Sum : Sum  Inputs=|++
  Sum1 : Sum  Inputs=+-
  Sum2 : Sum  Inputs=|++
  Switch : Switch  Criteria=u2 > Threshold
  Tf_Nm : Constant  Value=Tf_Nm
  Ts_s1 : InportShadow  Port=3
  Ts_s2 : InportShadow  Port=3
  Zero : Constant  Value=0
  dTheta_dt_rad_s : Outport
  Theta_rad : Outport  Port=2
  wires:
  Product1/1 -> Sum2/1
  Sum2/1 -> Delay1/1
  Delay1/1 -> Theta_rad/1, Sum2/2  "Theta_rad"
  Sum/1 -> Abs/1, Sign/1, Subtract/1  "new_momentum_excl_fricion"
  Product/1 -> Sum/1  "momentum_change_excl_friction"
  Ts_s/1 -> Product/2
  Sum1/1 -> Product/1  "Torque_excluding_friction"
  TB_Nm/1 -> Sum1/2
  TA_Nm/1 -> Sum1/1  "U_ist_uvw_V"
  Ts_s1/1 -> Product1/2
  Delay/1 -> InvMotorInertia_1_kgm2/1, Sum/2  "previous_momentum"
  Tf_Nm/1 -> Product2/1
  Ts_s2/1 -> Product2/2
  Product2/1 -> Product3/2, Relational Operator/2  "max_momentum_reduction_from_friction"
  Abs/1 -> Relational Operator/1
  Relational Operator/1 -> Switch/2
  Sign/1 -> Product3/1
  Product3/1 -> Subtract/2
  Subtract/1 -> Switch/1
  Zero/1 -> Switch/3
  Switch/1 -> Delay/1  "new_momentum"
  InvMotorInertia_1_kgm2/1 -> dTheta_dt_rad_s/1, Product1/1  "dTheta_dt_rad_s"

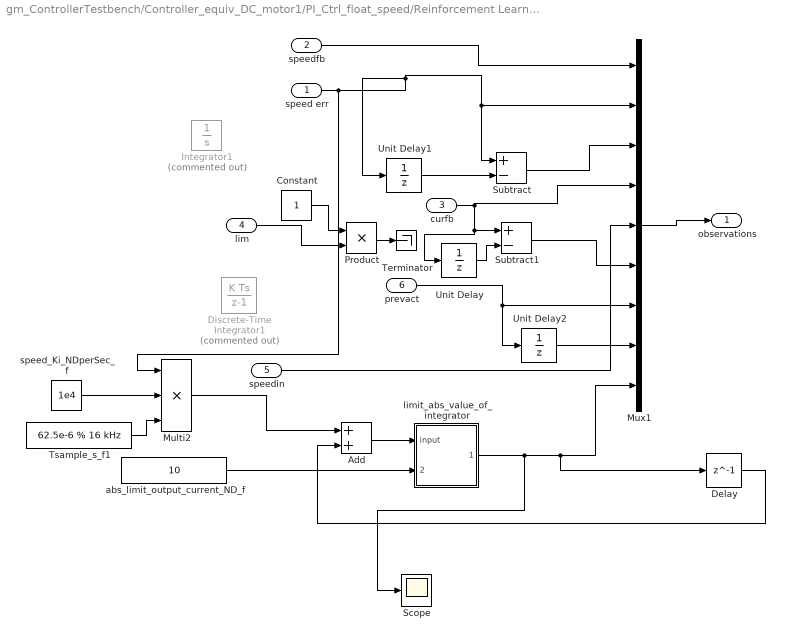
== system gm_ControllerTestbench/Controller_equiv_DC_motor1/PI_Ctrl_float_speed/Reinforcement Learning1/Observations ==
  speed err : Inport
  speedfb : Inport  Port=2
  curfb : Inport  Port=3
  lim : Inport  Port=4
  speedin : Inport  Port=5
  prevact : Inport  Port=6
  Add : Sum
  Constant : Constant
  Delay : Delay  DelayLength=1  InitialCondition=0
  Discrete-Time Integrator1 : DiscreteIntegrator  Commented=on  SampleTime=-1  ICPrevOutput=DiscIntNeverNeededParam  ICPrevScaledInput=DiscIntNeverNeededParam
  Integrator1 : Integrator  Commented=on
  Multi2 : Product  Inputs=***  RndMeth=Zero  SaturateOnIntegerOverflow=on
  Mux1 : Mux  Inputs=9
  Product : Product
  Scope : Scope
  Subtract : Sum  Inputs=+-
  Subtract1 : Sum  Inputs=+-
  Terminator : Terminator
  Tsample_s_f1 : Constant  Value=62.5e-6 % 16 kHz  OutDataTypeStr=double
  Unit Delay : UnitDelay  SampleTime=-1  HasFrameUpgradeWarning=on
  Unit Delay1 : UnitDelay  SampleTime=-1  HasFrameUpgradeWarning=on
  Unit Delay2 : UnitDelay  SampleTime=-1  HasFrameUpgradeWarning=on
  abs_limit_output_current_ND_f : Constant  Value=10  OutDataTypeStr=double
  limit_abs_value_of_integrator : Subsystem
  speed_Ki_NDperSec_f : Constant  Value=1e4  OutDataTypeStr=double
  observations : Outport  VectorParamsAs1DForOutWhenUnconnected=off
  wires:
  Mux1/1 -> observations/1
  speedfb/1 -> Mux1/1
  curfb/1 -> Subtract1/1, Unit Delay/1, Mux1/4
  Unit Delay1/1 -> Subtract/2
  Subtract/1 -> Mux1/3
  lim/1 -> Product/2
  Constant/1 -> Product/1
  prevact/1 -> Unit Delay2/1, Mux1/7
  speedin/1 -> Mux1/5
  Product/1 -> Terminator/1
  Unit Delay/1 -> Subtract1/2
  Subtract1/1 -> Mux1/6
  Unit Delay2/1 -> Mux1/8
  limit_abs_value_of_integrator/1(output) -> Scope/1, Delay/1, Mux1/9
  Delay/1 -> Add/2
  abs_limit_output_current_ND_f/1 -> limit_abs_value_of_integrator/2(abs_max)
  Add/1 -> limit_abs_value_of_integrator/1(input)
  speed err/1 -> Multi2/1, Subtract/1, Mux1/2, Unit Delay1/1
  speed_Ki_NDperSec_f/1 -> Multi2/2
  Tsample_s_f1/1 -> Multi2/3
  Multi2/1 -> Add/1

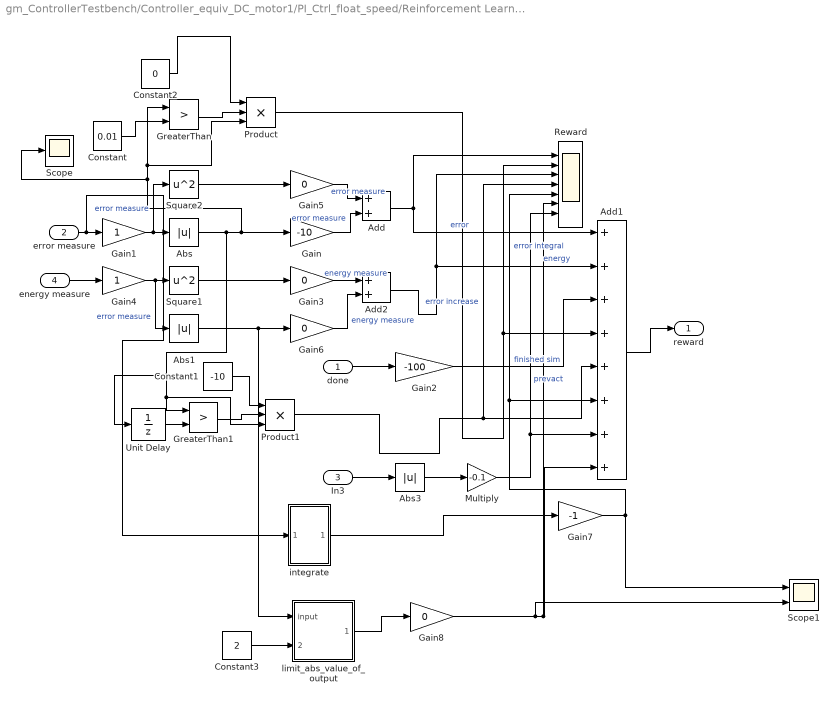
== system gm_ControllerTestbench/Controller_equiv_DC_motor1/PI_Ctrl_float_speed/Reinforcement Learning1/Reward ==
  done : Inport
  error measure : Inport  Port=2
  In3 : Inport  Port=3
  energy measure : Inport  Port=4
  Abs : Abs
  Abs1 : Abs
  Abs3 : Abs
  Add : Sum
  Add1 : Sum  Inputs=++++++++
  Add2 : Sum
  Constant : Constant  Value=0.01
  Constant1 : Constant  Value=-10
  Constant2 : Constant  Value=0
  Constant3 : Constant  Value=2
  Gain : Gain  Gain=-10
  Gain1 : Gain
  Gain2 : Gain  Gain=-100
  Gain{3,5..6,8} (4 alike) : Gain  Gain=0
  Gain4 : Gain
  Gain7 : Gain  Gain=-1
  GreaterThan : RelationalOperator  Operator=>  OutDataTypeStr=boolean  RndMeth=Simplest
  GreaterThan1 : RelationalOperator  Operator=>  OutDataTypeStr=boolean  RndMeth=Simplest
  Multiply : Gain  Gain=-0.1
  Product : Product  Inputs=3
  Product1 : Product  Inputs=3
  Reward : Scope  NumInputPorts=7
  Scope : Scope
  Scope1 : Scope  NumInputPorts=2
  Square1 : Math  Operator=square  SaturateOnIntegerOverflow=on
  Square2 : Math  Operator=square  SaturateOnIntegerOverflow=on
  Unit Delay : UnitDelay  SampleTime=-1  HasFrameUpgradeWarning=on
  integrate : Subsystem
  limit_abs_value_of_output : Subsystem
  reward : Outport  VectorParamsAs1DForOutWhenUnconnected=off
  wires:
  Add1/1 -> reward/1
  Gain2/1 -> Add1/3  "finished sim"
  done/1 -> Gain2/1
  Gain/1 -> Add/2  "error measure"
  Square1/1 -> Gain3/1
  error measure/1 -> integrate/1(In1), Gain1/1
  energy measure/1 -> Gain4/1
  Gain4/1 -> Abs1/1, Square1/1  "error measure"
  Gain1/1 -> Square2/1, Abs/1  "error measure"
  Square2/1 -> Gain5/1
  Gain5/1 -> Add/1  "error measure"
  Add/1 -> Reward/1, Add1/1  "error"
  Add2/1 -> Reward/3, Add1/2  "energy"
  Gain6/1 -> Add2/2  "energy measure"
  Gain3/1 -> Add2/1  "energy measure"
  Constant/1 -> GreaterThan/2
  GreaterThan/1 -> Product/2
  Product/1 -> Reward/2, Add1/4
  Constant2/1 -> Product/1
  Constant1/1 -> Product1/1
  GreaterThan1/1 -> Product1/2
  Abs/1 -> Unit Delay/1, Product1/3, GreaterThan1/1, Scope/1, Product/3, GreaterThan/1, Gain/1
  Unit Delay/1 -> GreaterThan1/2
  Product1/1 -> Reward/4, Add1/5  "error increase"
  Gain7/1 -> Reward/5, Add1/6, Scope1/1  "error integral"
  In3/1 -> Abs3/1
  Abs3/1 -> Multiply/1
  Multiply/1 -> Reward/7, Add1/7  "prevact"
  integrate/1(Out1) -> Gain7/1
  Gain8/1 -> Scope1/2, Reward/6, Add1/8
  limit_abs_value_of_output/1(output) -> Gain8/1
  Abs1/1 -> limit_abs_value_of_output/1(input), Gain6/1
  Constant3/1 -> limit_abs_value_of_output/2(abs_max)

== system gm_ControllerTestbench/Controller_equiv_DC_motor1/PI_Ctrl_float_speed/Reinforcement Learning1/Subsystem Reference2 ==
  Observations : Inport  OutDataTypeStr=fixdt(1, 18, 13)  PortDimensions=[9]  SampleTime=6.25e-05
  Hidden Layer (2 Neurons) : Subsystem
  Input Layer (4 Neurons) : Subsystem
  Output Layer (1 Neuron) : Subsystem
  bias 1 : Constant  Value=[-0.1662750244140625;0.28119659423828125;0.5211639404296875;0.779815673828125]  VectorParams1D=off  OutDataTypeStr=fixdt(1, 18, 17)  SampleTime=6.25e-05
  bias 2 : Constant  Value=[0.841403961181640625;0.13161468505859375]  VectorParams1D=off  OutDataTypeStr=fixdt(0, 18, 18)  SampleTime=6.25e-05
  bias 3 : Constant  Value=0.82561492919921875  VectorParams1D=off  OutDataTypeStr=fixdt(0, 18, 18)  SampleTime=6.25e-05
  delayMatch : Delay  DelayLength=double(4)  InitialCondition=0  SampleTime=6.25e-05
  t : Reshape  OutputDimensionality=Customize  OutputDimensions=[4,9]
  t1 : Reshape  OutputDimensionality=Customize  OutputDimensions=[2,4]
  weights 1 : Constant  Value=[0.236602783203125;-1.033660888671875;-0.512298583984375;1.162322998046875;0.122467041015625;3.169647216796875;0.64801025390625;-1.495513916015625;0.002838134765625;-0.022186279296875;-0.014801025390625;0.02215576171875;-0.066650390625;-0.238800048828125;-0.728363037109375;-0.100128173828125;0.351593017578125;1.0870361328125;-0.26544189453125;-0.3023681640625;-0.0662841796875;0.04595947265625;0.10540771484375;0.0155029296875;-0.086395263671875;-0.18035888671875;-0.29296875;-0.012298583984375;0.01885986328125;-0.009857177734375;-0.0196533203125;-0.003265380859375;0.011749267578125;0.02655029296875;0.0126953125;-0.149169921875]  VectorParams1D=off  OutDataTypeStr=fixdt(1, 18, 15)  SampleTime=6.25e-05
  weights 2 : Constant  Value=[-0.49188232421875;0.434814453125;-2.1717529296875;1.7066650390625;-0.46502685546875;0.5284423828125;1.285308837890625;-0.559051513671875]  VectorParams1D=off  OutDataTypeStr=fixdt(1, 18, 15)  SampleTime=6.25e-05
  weights 3 : Constant  Value=[-2.751373291015625 1.673797607421875]  VectorParams1D=off  OutDataTypeStr=fixdt(1, 18, 15)  SampleTime=6.25e-05
  Action : Outport
  wires:
  Observations/1 -> Input Layer (4 Neurons)/1(layer input)
  Hidden Layer (2 Neurons)/1(layer output) -> Output Layer (1 Neuron)/1(layer input)
  Input Layer (4 Neurons)/1(layer output) -> Hidden Layer (2 Neurons)/1(layer input)
  Output Layer (1 Neuron)/1(layer output) -> Action/1
  bias 1/1 -> Input Layer (4 Neurons)/3(bias vector)
  bias 2/1 -> Hidden Layer (2 Neurons)/3(bias vector)
  bias 3/1 -> Output Layer (1 Neuron)/3(bias vector1)
  t/1 -> Input Layer (4 Neurons)/2(weights matrix)
  delayMatch/1 -> Hidden Layer (2 Neurons)/2(weights matrix)
  weights 3/1 -> Output Layer (1 Neuron)/2(weights matrix1)
  weights 1/1 -> t/1
  weights 2/1 -> t1/1
  t1/1 -> delayMatch/1

== system gm_ControllerTestbench/PI Control Comparison/Controller_equiv_DC_motor/PI_Ctrl_float_speed/limit_abs_value_of_error_in ==
  input : Inport
  abs_max : Inport  Port=2
  CmpLT : RelationalOperator  Operator=<  OutDataTypeStr=boolean  RndMeth=Nearest
  CmpLT1 : RelationalOperator  OutDataTypeStr=boolean  RndMeth=Nearest
  Switch : Switch  Criteria=u2 ~= 0  Threshold=Position_PI_Limit  ZeroCross=off
  Switch1 : Switch  Criteria=u2 ~= 0  Threshold=I_max  ZeroCross=off
  Unary Minus : UnaryMinus
  output : Outport
  wires:
  Unary Minus/1 -> CmpLT/2, Switch1/1
  Switch1/1 -> output/1
  Switch/1 -> Switch1/3
  CmpLT/1 -> Switch1/2
  input/1 -> CmpLT/1, Switch/3, CmpLT1/1
  abs_max/1 -> Unary Minus/1, CmpLT1/2, Switch/1
  CmpLT1/1 -> Switch/2

== system gm_ControllerTestbench/PI Control Comparison/Controller_equiv_DC_motor/PI_Ctrl_float_speed/limit_abs_value_of_integrator ==
  input : Inport
  abs_max : Inport  Port=2
  CmpLT : RelationalOperator  Operator=<  OutDataTypeStr=boolean  RndMeth=Nearest
  CmpLT1 : RelationalOperator  OutDataTypeStr=boolean  RndMeth=Nearest
  Switch : Switch  Criteria=u2 ~= 0  Threshold=Position_PI_Limit  ZeroCross=off
  Switch1 : Switch  Criteria=u2 ~= 0  Threshold=I_max  ZeroCross=off
  Unary Minus : UnaryMinus
  output : Outport
  wires:
  CmpLT1/1 -> Switch/2
  abs_max/1 -> Switch/1, CmpLT1/2, Unary Minus/1
  input/1 -> CmpLT1/1, Switch/3, CmpLT/1
  CmpLT/1 -> Switch1/2
  Switch/1 -> Switch1/3
  Switch1/1 -> output/1
  Unary Minus/1 -> Switch1/1, CmpLT/2

== system gm_ControllerTestbench/PI Control Comparison/Controller_equiv_DC_motor/PI_Ctrl_float_speed/limit_abs_value_of_output ==
  input : Inport
  abs_max : Inport  Port=2
  CmpLT : RelationalOperator  Operator=<  OutDataTypeStr=boolean  RndMeth=Nearest
  CmpLT1 : RelationalOperator  OutDataTypeStr=boolean  RndMeth=Nearest
  Switch : Switch  Criteria=u2 ~= 0  Threshold=Position_PI_Limit  ZeroCross=off
  Switch1 : Switch  Criteria=u2 ~= 0  Threshold=I_max  ZeroCross=off
  Unary Minus : UnaryMinus
  output : Outport
  wires:
  Unary Minus/1 -> CmpLT/2, Switch1/1
  Switch1/1 -> output/1
  Switch/1 -> Switch1/3
  CmpLT/1 -> Switch1/2
  input/1 -> CmpLT/1, Switch/3, CmpLT1/1
  abs_max/1 -> Unary Minus/1, CmpLT1/2, Switch/1
  CmpLT1/1 -> Switch/2

== system gm_ControllerTestbench/PI Control Comparison/Controller_equiv_DC_motor/PI_Ctrl_float_speed1/limit_abs_value_of_error_in ==
  input : Inport
  abs_max : Inport  Port=2
  CmpLT : RelationalOperator  Operator=<  OutDataTypeStr=boolean  RndMeth=Nearest
  CmpLT1 : RelationalOperator  OutDataTypeStr=boolean  RndMeth=Nearest
  Switch : Switch  Criteria=u2 ~= 0  Threshold=Position_PI_Limit  ZeroCross=off
  Switch1 : Switch  Criteria=u2 ~= 0  Threshold=I_max  ZeroCross=off
  Unary Minus : UnaryMinus
  output : Outport
  wires:
  CmpLT1/1 -> Switch/2
  abs_max/1 -> Switch/1, CmpLT1/2, Unary Minus/1
  input/1 -> CmpLT1/1, Switch/3, CmpLT/1
  CmpLT/1 -> Switch1/2
  Switch/1 -> Switch1/3
  Switch1/1 -> output/1
  Unary Minus/1 -> Switch1/1, CmpLT/2

== system gm_ControllerTestbench/PI Control Comparison/Controller_equiv_DC_motor/PI_Ctrl_float_speed1/limit_abs_value_of_integrator ==
  input : Inport
  abs_max : Inport  Port=2
  CmpLT : RelationalOperator  Operator=<  OutDataTypeStr=boolean  RndMeth=Nearest
  CmpLT1 : RelationalOperator  OutDataTypeStr=boolean  RndMeth=Nearest
  Switch : Switch  Criteria=u2 ~= 0  Threshold=Position_PI_Limit  ZeroCross=off
  Switch1 : Switch  Criteria=u2 ~= 0  Threshold=I_max  ZeroCross=off
  Unary Minus : UnaryMinus
  output : Outport
  wires:
  Unary Minus/1 -> CmpLT/2, Switch1/1
  Switch1/1 -> output/1
  Switch/1 -> Switch1/3
  CmpLT/1 -> Switch1/2
  input/1 -> CmpLT/1, Switch/3, CmpLT1/1
  abs_max/1 -> Unary Minus/1, CmpLT1/2, Switch/1
  CmpLT1/1 -> Switch/2

== system gm_ControllerTestbench/PI Control Comparison/Controller_equiv_DC_motor/PI_Ctrl_float_speed1/limit_abs_value_of_output ==
  input : Inport
  abs_max : Inport  Port=2
  CmpLT : RelationalOperator  Operator=<  OutDataTypeStr=boolean  RndMeth=Nearest
  CmpLT1 : RelationalOperator  OutDataTypeStr=boolean  RndMeth=Nearest
  Switch : Switch  Criteria=u2 ~= 0  Threshold=Position_PI_Limit  ZeroCross=off
  Switch1 : Switch  Criteria=u2 ~= 0  Threshold=I_max  ZeroCross=off
  Unary Minus : UnaryMinus
  output : Outport
  wires:
  CmpLT1/1 -> Switch/2
  abs_max/1 -> Switch/1, CmpLT1/2, Unary Minus/1
  input/1 -> CmpLT1/1, Switch/3, CmpLT/1
  CmpLT/1 -> Switch1/2
  Switch/1 -> Switch1/3
  Switch1/1 -> output/1
  Unary Minus/1 -> Switch1/1, CmpLT/2

== system gm_ControllerTestbench/Controller_equiv_DC_motor1/PI_Ctrl_float_speed/Reinforcement Learning1/Observations/limit_abs_value_of_integrator ==
  input : Inport
  abs_max : Inport  Port=2
  CmpLT : RelationalOperator  Operator=<  OutDataTypeStr=boolean  RndMeth=Nearest
  CmpLT1 : RelationalOperator  OutDataTypeStr=boolean  RndMeth=Nearest
  Switch : Switch  Criteria=u2 ~= 0  Threshold=Position_PI_Limit  ZeroCross=off
  Switch1 : Switch  Criteria=u2 ~= 0  Threshold=I_max  ZeroCross=off
  Unary Minus : UnaryMinus
  output : Outport
  wires:
  CmpLT1/1 -> Switch/2
  abs_max/1 -> Switch/1, CmpLT1/2, Unary Minus/1
  input/1 -> CmpLT1/1, Switch/3, CmpLT/1
  CmpLT/1 -> Switch1/2
  Switch/1 -> Switch1/3
  Switch1/1 -> output/1
  Unary Minus/1 -> Switch1/1, CmpLT/2

== system gm_ControllerTestbench/Controller_equiv_DC_motor1/PI_Ctrl_float_speed/Reinforcement Learning1/Reward/integrate ==
  In1 : Inport
  Abs2 : Abs
  Add3 : Sum
  Delay : Delay  DelayLength=1  InitialCondition=0
  Multi2 : Product  Inputs=***  RndMeth=Zero  SaturateOnIntegerOverflow=on
  Tsample_s_f1 : Constant  Value=62.5e-6 % 16 kHz  OutDataTypeStr=double
  abs_limit_output_current_ND_f : Constant  Value=10  OutDataTypeStr=double
  limit_abs_value_of_integrator : Subsystem
  speed_Ki_NDperSec_f : Constant  Value=1e4  OutDataTypeStr=double
  Out1 : Outport
  wires:
  abs_limit_output_current_ND_f/1 -> limit_abs_value_of_integrator/2(abs_max)
  limit_abs_value_of_integrator/1(output) -> Abs2/1, Delay/1
  Add3/1 -> limit_abs_value_of_integrator/1(input)
  Abs2/1 -> Out1/1
  In1/1 -> Multi2/1
  Tsample_s_f1/1 -> Multi2/3
  Delay/1 -> Add3/2
  speed_Ki_NDperSec_f/1 -> Multi2/2
  Multi2/1 -> Add3/1

== system gm_ControllerTestbench/Controller_equiv_DC_motor1/PI_Ctrl_float_speed/Reinforcement Learning1/Reward/limit_abs_value_of_output ==
  input : Inport
  abs_max : Inport  Port=2
  CmpLT : RelationalOperator  Operator=<  OutDataTypeStr=boolean  RndMeth=Nearest
  CmpLT1 : RelationalOperator  OutDataTypeStr=boolean  RndMeth=Nearest
  Switch : Switch  Criteria=u2 ~= 0  Threshold=Position_PI_Limit  ZeroCross=off
  Switch1 : Switch  Criteria=u2 ~= 0  Threshold=I_max  ZeroCross=off
  Unary Minus : UnaryMinus
  output : Outport
  wires:
  Unary Minus/1 -> CmpLT/2, Switch1/1
  Switch1/1 -> output/1
  Switch/1 -> Switch1/3
  CmpLT/1 -> Switch1/2
  input/1 -> CmpLT/1, Switch/3, CmpLT1/1
  abs_max/1 -> Unary Minus/1, CmpLT1/2, Switch/1
  CmpLT1/1 -> Switch/2
